simulink model "CryoDetXray"  (R2016b)
settings: Solver=ode45  StartTime=0.0  StopTime=10e-5  MaxStep=Tclk/4  RelTol=1e-3
values from neighbouring files (symbols this model uses):
  Fclk = Fadc    (= 307200000)    [setupCryoFPGAxray.m]
  Tclk = 1/Fclk    (= 3.25520833333e-09)    [setupCryoFPGAxray.m]
undefined symbols (not defined in the file or in its folder): AXI4, Lite, lpf, Naxi, xlipgetpartsetting
libraries: xbsIndex_r4 x1091, CryoDetLib x68, simulink x4, hdlsllib x1
(part 4 of 8)

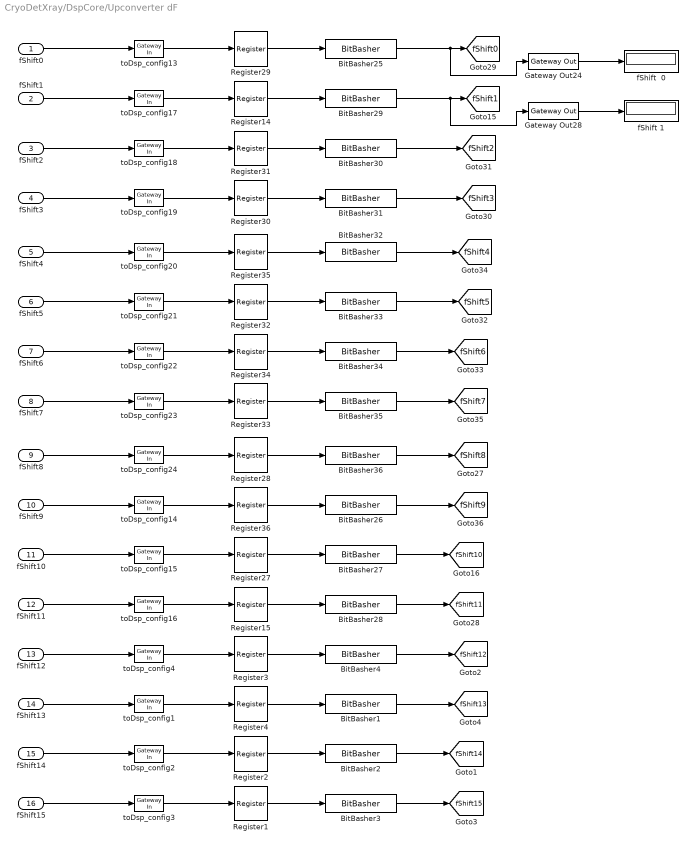
== system CryoDetXray/DspCore/Upconverter dF ==
  fShift0 : Inport
  fShift1 : Inport  Port=2
  fShift2 : Inport  Port=3
  fShift3 : Inport  Port=4
  fShift4 : Inport  Port=5
  fShift5 : Inport  Port=6
  fShift6 : Inport  Port=7
  fShift7 : Inport  Port=8
  fShift8 : Inport  Port=9
  fShift9 : Inport  Port=10
  fShift10 : Inport  Port=11
  fShift11 : Inport  Port=12
  fShift12 : Inport  Port=13
  fShift13 : Inport  Port=14
  fShift14 : Inport  Port=15
  fShift15 : Inport  Port=16
  BitBasher{1..4,25..36} (16 alike) : xbsIndex_r4/BitBasher  bitexpr=a={b[15:0]}  display_expr=on  sr_1=a  arith_type1=Unsigned  bin_pt1=16  sr_2=2  arith_type2=Unsigned  bin_pt2=0  sr_3=3  arith_type3=Unsigned  bin_pt3=0  sr_4=4  arith_type4=Unsigned  bin_pt4=0  dbl_ovrd=off  block_type=bitbasher
  Gateway Out24 : xbsIndex_r4/Gateway Out  inherit_from_input=on  hdl_port=off  rows=1  columns=1  UseAsDAC=off  DACChannel='1'  interface=None  automatic_assignment=on  address_offset=hex2dec('00')  intf_name=''  intf_description=''  timing_constraint=None  locs_specified=off  LOCs={}  io_standard={}  block_type=gatewayout
  Gateway Out28 : xbsIndex_r4/Gateway Out  inherit_from_input=on  hdl_port=off  rows=1  columns=1  UseAsDAC=off  DACChannel='1'  interface=None  automatic_assignment=on  address_offset=hex2dec('00')  intf_name=''  intf_description=''  timing_constraint=None  locs_specified=off  LOCs={}  io_standard={}  block_type=gatewayout
  Register{1..4,14..15,27..36} (16 alike) : xbsIndex_r4/Register  init=0  rst=off  en=off  dbl_ovrd=off  block_type=register
  fShift  0 : Display
  fShift 1 : Display
  toDsp_config1 : xbsIndex_r4/Gateway In  gui_display_data_type=Fixed-point  arith_type=Unsigned  n_bits=32  bin_pt=0  preci_type=Single  exp_width=8  frac_width=24  rows=1  columns=1  quantization=Truncate  overflow=Wrap  period=Tclk*Naxi  UseAsADC=off  ADCChannel='1'  interface=AXI4-Lite  automatic_assignment=off  address_offset=hex2dec('8B4')  intf_name=''  intf_description=''  default_value=0  timing_constraint=None  locs_specified=off  LOCs={}  io_standard={}  inherit_from_input=off  hdl_port=on  dbl_ovrd=off  block_type=gatewayin
  toDsp_config13 : xbsIndex_r4/Gateway In  gui_display_data_type=Fixed-point  arith_type=Unsigned  n_bits=32  bin_pt=0  preci_type=Single  exp_width=8  frac_width=24  rows=1  columns=1  quantization=Truncate  overflow=Wrap  period=Tclk*Naxi  UseAsADC=off  ADCChannel='1'  interface=AXI4-Lite  automatic_assignment=off  address_offset=hex2dec('880')  intf_name=''  intf_description=''  default_value=0  timing_constraint=None  locs_specified=off  LOCs={}  io_standard={}  inherit_from_input=off  hdl_port=on  dbl_ovrd=off  block_type=gatewayin
  toDsp_config14 : xbsIndex_r4/Gateway In  gui_display_data_type=Fixed-point  arith_type=Unsigned  n_bits=32  bin_pt=0  preci_type=Single  exp_width=8  frac_width=24  rows=1  columns=1  quantization=Truncate  overflow=Wrap  period=Tclk*Naxi  UseAsADC=off  ADCChannel='1'  interface=AXI4-Lite  automatic_assignment=off  address_offset=hex2dec('8A4')  intf_name=''  intf_description=''  default_value=0  timing_constraint=None  locs_specified=off  LOCs={}  io_standard={}  inherit_from_input=off  hdl_port=on  dbl_ovrd=off  block_type=gatewayin
  toDsp_config15 : xbsIndex_r4/Gateway In  gui_display_data_type=Fixed-point  arith_type=Unsigned  n_bits=32  bin_pt=0  preci_type=Single  exp_width=8  frac_width=24  rows=1  columns=1  quantization=Truncate  overflow=Wrap  period=Tclk*Naxi  UseAsADC=off  ADCChannel='1'  interface=AXI4-Lite  automatic_assignment=off  address_offset=hex2dec('8A8')  intf_name=''  intf_description=''  default_value=0  timing_constraint=None  locs_specified=off  LOCs={}  io_standard={}  inherit_from_input=off  hdl_port=on  dbl_ovrd=off  block_type=gatewayin
  toDsp_config16 : xbsIndex_r4/Gateway In  gui_display_data_type=Fixed-point  arith_type=Unsigned  n_bits=32  bin_pt=0  preci_type=Single  exp_width=8  frac_width=24  rows=1  columns=1  quantization=Truncate  overflow=Wrap  period=Tclk*Naxi  UseAsADC=off  ADCChannel='1'  interface=AXI4-Lite  automatic_assignment=off  address_offset=hex2dec('8AC')  intf_name=''  intf_description=''  default_value=0  timing_constraint=None  locs_specified=off  LOCs={}  io_standard={}  inherit_from_input=off  hdl_port=on  dbl_ovrd=off  block_type=gatewayin
  toDsp_config17 : xbsIndex_r4/Gateway In  gui_display_data_type=Fixed-point  arith_type=Unsigned  n_bits=32  bin_pt=0  preci_type=Single  exp_width=8  frac_width=24  rows=1  columns=1  quantization=Truncate  overflow=Wrap  period=Tclk*Naxi  UseAsADC=off  ADCChannel='1'  interface=AXI4-Lite  automatic_assignment=off  address_offset=hex2dec('884')  intf_name=''  intf_description=''  default_value=0  timing_constraint=None  locs_specified=off  LOCs={}  io_standard={}  inherit_from_input=off  hdl_port=on  dbl_ovrd=off  block_type=gatewayin
  toDsp_config18 : xbsIndex_r4/Gateway In  gui_display_data_type=Fixed-point  arith_type=Unsigned  n_bits=32  bin_pt=0  preci_type=Single  exp_width=8  frac_width=24  rows=1  columns=1  quantization=Truncate  overflow=Wrap  period=Tclk*Naxi  UseAsADC=off  ADCChannel='1'  interface=AXI4-Lite  automatic_assignment=off  address_offset=hex2dec('888')  intf_name=''  intf_description=''  default_value=0  timing_constraint=None  locs_specified=off  LOCs={}  io_standard={}  inherit_from_input=off  hdl_port=on  dbl_ovrd=off  block_type=gatewayin
  toDsp_config19 : xbsIndex_r4/Gateway In  gui_display_data_type=Fixed-point  arith_type=Unsigned  n_bits=32  bin_pt=0  preci_type=Single  exp_width=8  frac_width=24  rows=1  columns=1  quantization=Truncate  overflow=Wrap  period=Tclk*Naxi  UseAsADC=off  ADCChannel='1'  interface=AXI4-Lite  automatic_assignment=off  address_offset=hex2dec('88c')  intf_name=''  intf_description=''  default_value=0  timing_constraint=None  locs_specified=off  LOCs={}  io_standard={}  inherit_from_input=off  hdl_port=on  dbl_ovrd=off  block_type=gatewayin
  toDsp_config2 : xbsIndex_r4/Gateway In  gui_display_data_type=Fixed-point  arith_type=Unsigned  n_bits=32  bin_pt=0  preci_type=Single  exp_width=8  frac_width=24  rows=1  columns=1  quantization=Truncate  overflow=Wrap  period=Tclk*Naxi  UseAsADC=off  ADCChannel='1'  interface=AXI4-Lite  automatic_assignment=off  address_offset=hex2dec('8B8')  intf_name=''  intf_description=''  default_value=0  timing_constraint=None  locs_specified=off  LOCs={}  io_standard={}  inherit_from_input=off  hdl_port=on  dbl_ovrd=off  block_type=gatewayin
  toDsp_config20 : xbsIndex_r4/Gateway In  gui_display_data_type=Fixed-point  arith_type=Unsigned  n_bits=32  bin_pt=0  preci_type=Single  exp_width=8  frac_width=24  rows=1  columns=1  quantization=Truncate  overflow=Wrap  period=Tclk*Naxi  UseAsADC=off  ADCChannel='1'  interface=AXI4-Lite  automatic_assignment=off  address_offset=hex2dec('890')  intf_name=''  intf_description=''  default_value=0  timing_constraint=None  locs_specified=off  LOCs={}  io_standard={}  inherit_from_input=off  hdl_port=on  dbl_ovrd=off  block_type=gatewayin
  toDsp_config21 : xbsIndex_r4/Gateway In  gui_display_data_type=Fixed-point  arith_type=Unsigned  n_bits=32  bin_pt=0  preci_type=Single  exp_width=8  frac_width=24  rows=1  columns=1  quantization=Truncate  overflow=Wrap  period=Tclk*Naxi  UseAsADC=off  ADCChannel='1'  interface=AXI4-Lite  automatic_assignment=off  address_offset=hex2dec('894')  intf_name=''  intf_description=''  default_value=0  timing_constraint=None  locs_specified=off  LOCs={}  io_standard={}  inherit_from_input=off  hdl_port=on  dbl_ovrd=off  block_type=gatewayin
  toDsp_config22 : xbsIndex_r4/Gateway In  gui_display_data_type=Fixed-point  arith_type=Unsigned  n_bits=32  bin_pt=0  preci_type=Single  exp_width=8  frac_width=24  rows=1  columns=1  quantization=Truncate  overflow=Wrap  period=Tclk*Naxi  UseAsADC=off  ADCChannel='1'  interface=AXI4-Lite  automatic_assignment=off  address_offset=hex2dec('898')  intf_name=''  intf_description=''  default_value=0  timing_constraint=None  locs_specified=off  LOCs={}  io_standard={}  inherit_from_input=off  hdl_port=on  dbl_ovrd=off  block_type=gatewayin
  toDsp_config23 : xbsIndex_r4/Gateway In  gui_display_data_type=Fixed-point  arith_type=Unsigned  n_bits=32  bin_pt=0  preci_type=Single  exp_width=8  frac_width=24  rows=1  columns=1  quantization=Truncate  overflow=Wrap  period=Tclk*Naxi  UseAsADC=off  ADCChannel='1'  interface=AXI4-Lite  automatic_assignment=off  address_offset=hex2dec('89c')  intf_name=''  intf_description=''  default_value=0  timing_constraint=None  locs_specified=off  LOCs={}  io_standard={}  inherit_from_input=off  hdl_port=on  dbl_ovrd=off  block_type=gatewayin
  toDsp_config24 : xbsIndex_r4/Gateway In  gui_display_data_type=Fixed-point  arith_type=Unsigned  n_bits=32  bin_pt=0  preci_type=Single  exp_width=8  frac_width=24  rows=1  columns=1  quantization=Truncate  overflow=Wrap  period=Tclk*Naxi  UseAsADC=off  ADCChannel='1'  interface=AXI4-Lite  automatic_assignment=off  address_offset=hex2dec('8A0')  intf_name=''  intf_description=''  default_value=0  timing_constraint=None  locs_specified=off  LOCs={}  io_standard={}  inherit_from_input=off  hdl_port=on  dbl_ovrd=off  block_type=gatewayin
  toDsp_config3 : xbsIndex_r4/Gateway In  gui_display_data_type=Fixed-point  arith_type=Unsigned  n_bits=32  bin_pt=0  preci_type=Single  exp_width=8  frac_width=24  rows=1  columns=1  quantization=Truncate  overflow=Wrap  period=Tclk*Naxi  UseAsADC=off  ADCChannel='1'  interface=AXI4-Lite  automatic_assignment=off  address_offset=hex2dec('8BC')  intf_name=''  intf_description=''  default_value=0  timing_constraint=None  locs_specified=off  LOCs={}  io_standard={}  inherit_from_input=off  hdl_port=on  dbl_ovrd=off  block_type=gatewayin
  toDsp_config4 : xbsIndex_r4/Gateway In  gui_display_data_type=Fixed-point  arith_type=Unsigned  n_bits=32  bin_pt=0  preci_type=Single  exp_width=8  frac_width=24  rows=1  columns=1  quantization=Truncate  overflow=Wrap  period=Tclk*Naxi  UseAsADC=off  ADCChannel='1'  interface=AXI4-Lite  automatic_assignment=off  address_offset=hex2dec('8B0')  intf_name=''  intf_description=''  default_value=0  timing_constraint=None  locs_specified=off  LOCs={}  io_standard={}  inherit_from_input=off  hdl_port=on  dbl_ovrd=off  block_type=gatewayin
  tag scope: fShift0=global, fShift10=global, fShift11=global, fShift12=global, fShift13=global, fShift14=global, fShift15=global, fShift1=global, fShift2=global, fShift3=global, fShift4=global, fShift5=global, fShift6=global, fShift7=global, fShift8=global, fShift9=global
  wires:
  toDsp_config13/1 -> Register29/1
  fShift10/1 -> toDsp_config15/1
  toDsp_config15/1 -> Register27/1
  Register32/1 -> BitBasher33/1
  BitBasher28/1 -> [fShift11]
  Register15/1 -> BitBasher28/1
  toDsp_config21/1 -> Register32/1
  BitBasher32/1 -> [fShift4]
  Register27/1 -> BitBasher27/1
  BitBasher27/1 -> [fShift10]
  fShift0/1 -> toDsp_config13/1
  fShift7/1 -> toDsp_config23/1
  toDsp_config23/1 -> Register33/1
  Gateway Out24/1 -> fShift  0/1
  Register30/1 -> BitBasher31/1
  BitBasher30/1 -> [fShift2]
  BitBasher31/1 -> [fShift3]
  Register33/1 -> BitBasher35/1
  Register36/1 -> BitBasher26/1
  fShift2/1 -> toDsp_config18/1
  toDsp_config18/1 -> Register31/1
  BitBasher29/1 -> Gateway Out28/1, [fShift1]
  BitBasher34/1 -> [fShift6]
  toDsp_config17/1 -> Register14/1
  fShift1/1 -> toDsp_config17/1
  Register28/1 -> BitBasher36/1
  BitBasher33/1 -> [fShift5]
  BitBasher35/1 -> [fShift7]
  BitBasher25/1 -> Gateway Out24/1, [fShift0]
  fShift5/1 -> toDsp_config21/1
  BitBasher36/1 -> [fShift8]
  Register34/1 -> BitBasher34/1
  BitBasher26/1 -> [fShift9]
  fShift8/1 -> toDsp_config24/1
  toDsp_config24/1 -> Register28/1
  fShift6/1 -> toDsp_config22/1
  toDsp_config22/1 -> Register34/1
  fShift11/1 -> toDsp_config16/1
  toDsp_config16/1 -> Register15/1
  fShift9/1 -> toDsp_config14/1
  toDsp_config14/1 -> Register36/1
  Register29/1 -> BitBasher25/1
  Register35/1 -> BitBasher32/1
  toDsp_config20/1 -> Register35/1
  fShift4/1 -> toDsp_config20/1
  Register14/1 -> BitBasher29/1
  Gateway Out28/1 -> fShift 1/1
  Register31/1 -> BitBasher30/1
  fShift3/1 -> toDsp_config19/1
  toDsp_config19/1 -> Register30/1
  fShift14/1 -> toDsp_config2/1
  toDsp_config2/1 -> Register2/1
  BitBasher3/1 -> [fShift15]
  Register1/1 -> BitBasher3/1
  Register2/1 -> BitBasher2/1
  BitBasher2/1 -> [fShift14]
  Register4/1 -> BitBasher1/1
  Register3/1 -> BitBasher4/1
  BitBasher4/1 -> [fShift12]
  BitBasher1/1 -> [fShift13]
  fShift12/1 -> toDsp_config4/1
  toDsp_config4/1 -> Register3/1
  fShift15/1 -> toDsp_config3/1
  toDsp_config3/1 -> Register1/1
  fShift13/1 -> toDsp_config1/1
  toDsp_config1/1 -> Register4/1

== system CryoDetXray/DspCore/eta input ==
  note: Punt for now on ch 3-11
  Re eta 0 : Inport
  Im eta 0 : Inport  Port=2
  Re eta 1 : Inport  Port=3
  Im eta 1 : Inport  Port=4
  Re eta 2 : Inport  Port=5
  Im eta 2 : Inport  Port=6
  Constant : xbsIndex_r4/Constant  const=0  gui_display_data_type=Fixed-point  arith_type=Signed (2's comp)  n_bits=32  bin_pt=14  preci_type=Single  exp_width=8  frac_width=24  explicit_period=off  period=1  equ=P=C  opselect=C  inp2=PCIN>>17  opr=+  inp1=P  carry=CIN  dbl_ovrd=off  block_type=constant
  Gateway Out{36..41} (6 alike) : xbsIndex_r4/Gateway Out  inherit_from_input=on  hdl_port=off  rows=1  columns=1  UseAsDAC=off  DACChannel='1'  interface=None  automatic_assignment=on  address_offset=hex2dec('00')  intf_name=''  intf_description=''  timing_constraint=None  locs_specified=off  LOCs={}  io_standard={}  block_type=gatewayout
  Register{37..42} (6 alike) : xbsIndex_r4/Register  init=0  rst=off  en=off  dbl_ovrd=off  block_type=register
  im eta 0 : Display
  im eta 1 : Display
  im eta 2 : Display
  re eta 0 : Display
  re eta 1 : Display
  re eta 2 : Display
  toDsp_config25 : xbsIndex_r4/Gateway In  gui_display_data_type=Fixed-point  arith_type="Signed  (2's comp)"  n_bits=32  bin_pt=14  preci_type=Single  exp_width=8  frac_width=24  rows=1  columns=1  quantization=Truncate  overflow=Wrap  period=Tclk*Naxi  UseAsADC=off  ADCChannel='1'  interface=AXI4-Lite  automatic_assignment=off  address_offset=hex2dec('C00')  intf_name=''  intf_description=''  default_value=0  timing_constraint=None  locs_specified=off  LOCs={}  io_standard={}  inherit_from_input=off  hdl_port=on  dbl_ovrd=off  block_type=gatewayin
  toDsp_config26 : xbsIndex_r4/Gateway In  gui_display_data_type=Fixed-point  arith_type="Signed  (2's comp)"  n_bits=32  bin_pt=14  preci_type=Single  exp_width=8  frac_width=24  rows=1  columns=1  quantization=Truncate  overflow=Wrap  period=Tclk*Naxi  UseAsADC=off  ADCChannel='1'  interface=AXI4-Lite  automatic_assignment=off  address_offset=hex2dec('D00')  intf_name=''  intf_description=''  default_value=0  timing_constraint=None  locs_specified=off  LOCs={}  io_standard={}  inherit_from_input=off  hdl_port=on  dbl_ovrd=off  block_type=gatewayin
  toDsp_config27 : xbsIndex_r4/Gateway In  gui_display_data_type=Fixed-point  arith_type="Signed  (2's comp)"  n_bits=32  bin_pt=14  preci_type=Single  exp_width=8  frac_width=24  rows=1  columns=1  quantization=Truncate  overflow=Wrap  period=Tclk*Naxi  UseAsADC=off  ADCChannel='1'  interface=AXI4-Lite  automatic_assignment=off  address_offset=hex2dec('C04')  intf_name=''  intf_description=''  default_value=0  timing_constraint=None  locs_specified=off  LOCs={}  io_standard={}  inherit_from_input=off  hdl_port=on  dbl_ovrd=off  block_type=gatewayin
  toDsp_config28 : xbsIndex_r4/Gateway In  gui_display_data_type=Fixed-point  arith_type="Signed  (2's comp)"  n_bits=32  bin_pt=14  preci_type=Single  exp_width=8  frac_width=24  rows=1  columns=1  quantization=Truncate  overflow=Wrap  period=Tclk*Naxi  UseAsADC=off  ADCChannel='1'  interface=AXI4-Lite  automatic_assignment=off  address_offset=hex2dec('D04')  intf_name=''  intf_description=''  default_value=0  timing_constraint=None  locs_specified=off  LOCs={}  io_standard={}  inherit_from_input=off  hdl_port=on  dbl_ovrd=off  block_type=gatewayin
  toDsp_config29 : xbsIndex_r4/Gateway In  gui_display_data_type=Fixed-point  arith_type="Signed  (2's comp)"  n_bits=32  bin_pt=14  preci_type=Single  exp_width=8  frac_width=24  rows=1  columns=1  quantization=Truncate  overflow=Wrap  period=Tclk*Naxi  UseAsADC=off  ADCChannel='1'  interface=AXI4-Lite  automatic_assignment=off  address_offset=hex2dec('C08')  intf_name=''  intf_description=''  default_value=0  timing_constraint=None  locs_specified=off  LOCs={}  io_standard={}  inherit_from_input=off  hdl_port=on  dbl_ovrd=off  block_type=gatewayin
  toDsp_config30 : xbsIndex_r4/Gateway In  gui_display_data_type=Fixed-point  arith_type="Signed  (2's comp)"  n_bits=32  bin_pt=14  preci_type=Single  exp_width=8  frac_width=24  rows=1  columns=1  quantization=Truncate  overflow=Wrap  period=Tclk*Naxi  UseAsADC=off  ADCChannel='1'  interface=AXI4-Lite  automatic_assignment=off  address_offset=hex2dec('D08')  intf_name=''  intf_description=''  default_value=0  timing_constraint=None  locs_specified=off  LOCs={}  io_standard={}  inherit_from_input=off  hdl_port=on  dbl_ovrd=off  block_type=gatewayin
  tag scope: imEta0=global, imEta10=global, imEta11=global, imEta12=global, imEta13=global, imEta14=global, imEta15=global, imEta1=global, imEta2=global, imEta3=global, imEta4=global, imEta5=global, imEta6=global, imEta7=global, imEta8=global, imEta9=global, reEta0=global, reEta10=global, reEta11=global, reEta12=global, reEta13=global, reEta14=global, reEta15=global, reEta1=global, reEta2=global, reEta3=global, reEta4=global, reEta5=global, reEta6=global, reEta7=global, reEta8=global, reEta9=global
  wires:
  toDsp_config28/1 -> Register39/1
  Im eta 1/1 -> toDsp_config28/1
  Register40/1 -> Gateway Out38/1, [reEta1]
  Gateway Out39/1 -> im eta 1/1
  Re eta 2/1 -> toDsp_config29/1
  Gateway Out40/1 -> re eta 2/1
  Register41/1 -> Gateway Out41/1, [imEta2]
  toDsp_config30/1 -> Register41/1
  Im eta 2/1 -> toDsp_config30/1
  toDsp_config27/1 -> Register40/1
  Re eta 1/1 -> toDsp_config27/1
  Gateway Out38/1 -> re eta 1/1
  Register39/1 -> Gateway Out39/1, [imEta1]
  Register42/1 -> Gateway Out40/1, [reEta2]
  Gateway Out41/1 -> im eta 2/1
  toDsp_config29/1 -> Register42/1
  Constant/1 -> [reEta4], [reEta5], [reEta6], [reEta7], [reEta8], [reEta9], [imEta9], [imEta10], [imEta12], [imEta13], [imEta14], [imEta15], [imEta11], [imEta8], [imEta7], [imEta6], [imEta5], [imEta4], [imEta3], [reEta15], [reEta14], [reEta13], [reEta12], [reEta11], [reEta10], [reEta3]
  toDsp_config25/1 -> Register38/1
  Re eta 0/1 -> toDsp_config25/1
  Gateway Out36/1 -> re eta 0/1
  Register37/1 -> Gateway Out37/1, [imEta0]
  toDsp_config26/1 -> Register37/1
  Im eta 0/1 -> toDsp_config26/1
  Register38/1 -> Gateway Out36/1, [reEta0]
  Gateway Out37/1 -> im eta 0/1

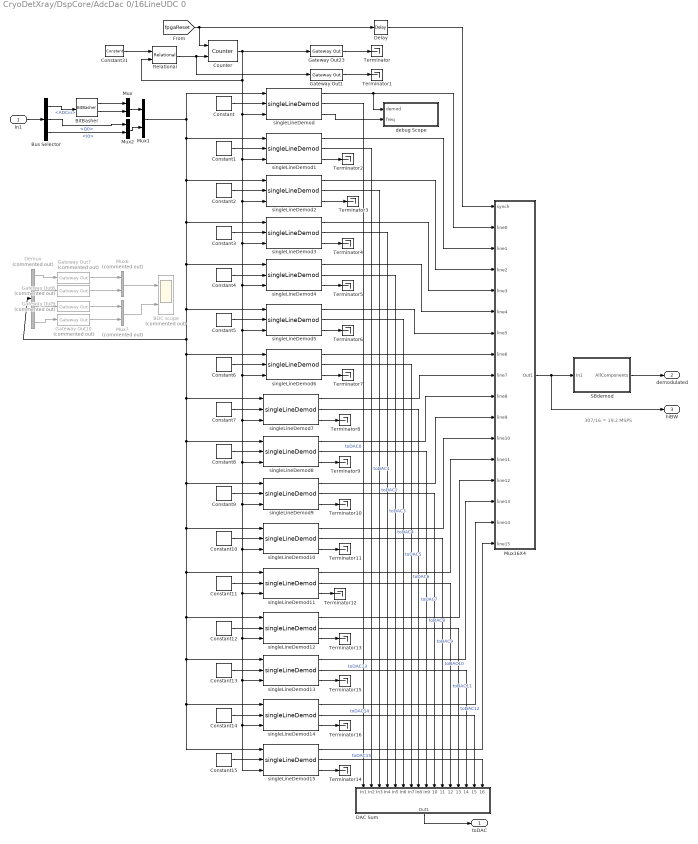
== system CryoDetXray/DspCore/AdcDac 0/16LineUDC 0 ==
  note: 307/16 = 19.2 MSPS
  In1 : Inport
  BDC scope : Scope  Commented=on  NumInputPorts=2
  BitBasher : xbsIndex_r4/BitBasher  bitexpr=|  display_expr=off  sr_1=Q  arith_type1="Signed  (2's comp)"  bin_pt1=15  sr_2=I  arith_type2="Signed  (2's comp)"  bin_pt2=15  sr_3=I  arith_type3=Unsigned  bin_pt3=0  sr_4=4  arith_type4=Unsigned  bin_pt4=0  dbl_ovrd=off  block_type=bitbasher
      | Q = {adc[15:0]}
      | I = {adc[31:16]}
  Bus Selector : BusSelector  OutputSignals=ADCin,refDel.Q0,refDel.I0
  Constant : xbsIndex_r4/Constant  const=0  gui_display_data_type=Fixed-point  arith_type=Unsigned  n_bits=4  bin_pt=0  preci_type=Single  exp_width=8  frac_width=24  explicit_period=off  period=1  equ=P=C  opselect=C  inp2=PCIN>>17  opr=+  inp1=P  carry=CIN  dbl_ovrd=off  block_type=constant
  Constant1 : xbsIndex_r4/Constant  const=1  gui_display_data_type=Fixed-point  arith_type=Unsigned  n_bits=4  bin_pt=0  preci_type=Single  exp_width=8  frac_width=24  explicit_period=off  period=1  equ=P=C  opselect=C  inp2=PCIN>>17  opr=+  inp1=P  carry=CIN  dbl_ovrd=off  block_type=constant
  Constant10 : xbsIndex_r4/Constant  const=10  gui_display_data_type=Fixed-point  arith_type=Unsigned  n_bits=4  bin_pt=0  preci_type=Single  exp_width=8  frac_width=24  explicit_period=off  period=1  equ=P=C  opselect=C  inp2=PCIN>>17  opr=+  inp1=P  carry=CIN  dbl_ovrd=off  block_type=constant
  Constant11 : xbsIndex_r4/Constant  const=11  gui_display_data_type=Fixed-point  arith_type=Unsigned  n_bits=4  bin_pt=0  preci_type=Single  exp_width=8  frac_width=24  explicit_period=off  period=1  equ=P=C  opselect=C  inp2=PCIN>>17  opr=+  inp1=P  carry=CIN  dbl_ovrd=off  block_type=constant
  Constant12 : xbsIndex_r4/Constant  const=12  gui_display_data_type=Fixed-point  arith_type=Unsigned  n_bits=4  bin_pt=0  preci_type=Single  exp_width=8  frac_width=24  explicit_period=off  period=1  equ=P=C  opselect=C  inp2=PCIN>>17  opr=+  inp1=P  carry=CIN  dbl_ovrd=off  block_type=constant
  Constant13 : xbsIndex_r4/Constant  const=13  gui_display_data_type=Fixed-point  arith_type=Unsigned  n_bits=4  bin_pt=0  preci_type=Single  exp_width=8  frac_width=24  explicit_period=off  period=1  equ=P=C  opselect=C  inp2=PCIN>>17  opr=+  inp1=P  carry=CIN  dbl_ovrd=off  block_type=constant
  Constant14 : xbsIndex_r4/Constant  const=14  gui_display_data_type=Fixed-point  arith_type=Unsigned  n_bits=4  bin_pt=0  preci_type=Single  exp_width=8  frac_width=24  explicit_period=off  period=1  equ=P=C  opselect=C  inp2=PCIN>>17  opr=+  inp1=P  carry=CIN  dbl_ovrd=off  block_type=constant
  Constant15 : xbsIndex_r4/Constant  const=15  gui_display_data_type=Fixed-point  arith_type=Unsigned  n_bits=4  bin_pt=0  preci_type=Single  exp_width=8  frac_width=24  explicit_period=off  period=1  equ=P=C  opselect=C  inp2=PCIN>>17  opr=+  inp1=P  carry=CIN  dbl_ovrd=off  block_type=constant
  Constant2 : xbsIndex_r4/Constant  const=2  gui_display_data_type=Fixed-point  arith_type=Unsigned  n_bits=4  bin_pt=0  preci_type=Single  exp_width=8  frac_width=24  explicit_period=off  period=1  equ=P=C  opselect=C  inp2=PCIN>>17  opr=+  inp1=P  carry=CIN  dbl_ovrd=off  block_type=constant
  Constant3 : xbsIndex_r4/Constant  const=3  gui_display_data_type=Fixed-point  arith_type=Unsigned  n_bits=4  bin_pt=0  preci_type=Single  exp_width=8  frac_width=24  explicit_period=off  period=1  equ=P=C  opselect=C  inp2=PCIN>>17  opr=+  inp1=P  carry=CIN  dbl_ovrd=off  block_type=constant
  Constant31 : xbsIndex_r4/Constant  const=31  gui_display_data_type=Fixed-point  arith_type=Unsigned  n_bits=5  bin_pt=0  preci_type=Single  exp_width=8  frac_width=24  explicit_period=off  period=1  equ=P=C  opselect=C  inp2=PCIN>>17  opr=+  inp1=P  carry=CIN  dbl_ovrd=off  block_type=constant
  Constant4 : xbsIndex_r4/Constant  const=4  gui_display_data_type=Fixed-point  arith_type=Unsigned  n_bits=4  bin_pt=0  preci_type=Single  exp_width=8  frac_width=24  explicit_period=off  period=1  equ=P=C  opselect=C  inp2=PCIN>>17  opr=+  inp1=P  carry=CIN  dbl_ovrd=off  block_type=constant
  Constant5 : xbsIndex_r4/Constant  const=5  gui_display_data_type=Fixed-point  arith_type=Unsigned  n_bits=4  bin_pt=0  preci_type=Single  exp_width=8  frac_width=24  explicit_period=off  period=1  equ=P=C  opselect=C  inp2=PCIN>>17  opr=+  inp1=P  carry=CIN  dbl_ovrd=off  block_type=constant
  Constant6 : xbsIndex_r4/Constant  const=6  gui_display_data_type=Fixed-point  arith_type=Unsigned  n_bits=4  bin_pt=0  preci_type=Single  exp_width=8  frac_width=24  explicit_period=off  period=1  equ=P=C  opselect=C  inp2=PCIN>>17  opr=+  inp1=P  carry=CIN  dbl_ovrd=off  block_type=constant
  Constant7 : xbsIndex_r4/Constant  const=7  gui_display_data_type=Fixed-point  arith_type=Unsigned  n_bits=4  bin_pt=0  preci_type=Single  exp_width=8  frac_width=24  explicit_period=off  period=1  equ=P=C  opselect=C  inp2=PCIN>>17  opr=+  inp1=P  carry=CIN  dbl_ovrd=off  block_type=constant
  Constant8 : xbsIndex_r4/Constant  const=8  gui_display_data_type=Fixed-point  arith_type=Unsigned  n_bits=4  bin_pt=0  preci_type=Single  exp_width=8  frac_width=24  explicit_period=off  period=1  equ=P=C  opselect=C  inp2=PCIN>>17  opr=+  inp1=P  carry=CIN  dbl_ovrd=off  block_type=constant
  Constant9 : xbsIndex_r4/Constant  const=9  gui_display_data_type=Fixed-point  arith_type=Unsigned  n_bits=4  bin_pt=0  preci_type=Single  exp_width=8  frac_width=24  explicit_period=off  period=1  equ=P=C  opselect=C  inp2=PCIN>>17  opr=+  inp1=P  carry=CIN  dbl_ovrd=off  block_type=constant
  Counter : xbsIndex_r4/Counter  cnt_type=Count Limited  cnt_to=31  operation=Up  start_count=0  cnt_by_val=1  arith_type=Unsigned  n_bits=5  bin_pt=0  load_pin=off  rst=on  en=on  explicit_period=off  period=Tclk  use_behavioral_HDL=off  implementation=Fabric  dbl_ovrd=off  block_type=counter
  DAC Sum : Subsystem
  Delay : xbsIndex_r4/Delay  rst=off  infoeditControl=Selection of Reset will increase slice count due to use of real FFs and instead of SRLs  en=off  latency=6  reg_retiming=off  dbl_ovrd=off  block_type=delay
  Demux : Demux  Commented=on
  Gateway Out1 : xbsIndex_r4/Gateway Out  inherit_from_input=off  hdl_port=off  rows=1  columns=1  UseAsDAC=off  DACChannel='1'  interface=None  automatic_assignment=on  address_offset=hex2dec('00')  intf_name=''  intf_description=''  timing_constraint=None  locs_specified=off  LOCs={}  io_standard={}  block_type=gatewayout
  Gateway Out{7..10} (4 alike) : xbsIndex_r4/Gateway Out  Commented=on  inherit_from_input=off  hdl_port=off  rows=1  columns=1  UseAsDAC=off  DACChannel='1'  interface=None  automatic_assignment=on  address_offset=hex2dec('00')  intf_name=''  intf_description=''  timing_constraint=None  locs_specified=off  LOCs={}  io_standard={}  block_type=gatewayout
  Gateway Out23 : xbsIndex_r4/Gateway Out  inherit_from_input=off  hdl_port=off  rows=1  columns=1  UseAsDAC=off  DACChannel='1'  interface=None  automatic_assignment=on  address_offset=hex2dec('00')  intf_name=''  intf_description=''  timing_constraint=None  locs_specified=off  LOCs={}  io_standard={}  block_type=gatewayout
  Mux : Mux  Inputs=2
  Mux1 : Mux  Inputs=2
  Mux16X4 : Subsystem
  Mux2 : Mux  Inputs=2
  Mux6 : Mux  Commented=on  Inputs=2
  Mux7 : Mux  Commented=on  Inputs=2
  Relational : xbsIndex_r4/Relational  mode=a!=b  op_type=Bool  en=off  latency=0  dbl_ovrd=off  block_type=relational
  SBdemod : Subsystem
  Terminator{,1..16} (17 alike) : Terminator
  debug Scope : Subsystem
  singleLineDemod{,1..15} (16 alike) : CryoDetLib/singleLineDemod
  toDAC : Outport
  demodulated : Outport  Port=2
  hiBW : Outport  Port=3
  wires:
  [fpgaReset] -> Counter/1, Delay/1
  singleLineDemod7/1 -> Mux16X4/9(line7)
  singleLineDemod6/1 -> Mux16X4/8(line6)
  singleLineDemod5/1 -> Mux16X4/7(line5)
  singleLineDemod4/1 -> Mux16X4/6(line4)
  singleLineDemod3/1 -> Mux16X4/5(line3)
  singleLineDemod2/1 -> Mux16X4/4(line2)
  Mux16X4/1(Out1) -> hiBW/1, SBdemod/1(In1)
  singleLineDemod1/1 -> Mux16X4/3(line1)
  singleLineDemod/1 -> debug Scope/1(demod), Mux16X4/2(line0)
  singleLineDemod8/1 -> Mux16X4/10(line8)
  singleLineDemod9/1 -> Mux16X4/11(line9)
  singleLineDemod10/1 -> Mux16X4/12(line10)
  singleLineDemod11/1 -> Mux16X4/13(line11)
  singleLineDemod11/2 -> DAC Sum/12(In12)  "toDAC11"
  singleLineDemod10/2 -> DAC Sum/11(In11)  "toDAC10"
  singleLineDemod9/2 -> DAC Sum/10(In10)  "toDAC9"
  singleLineDemod8/2 -> DAC Sum/9(In9)  "toDAC8"
  singleLineDemod7/2 -> DAC Sum/8(In8)  "toDAC7"
  singleLineDemod6/2 -> DAC Sum/7(In7)  "toDAC6"
  singleLineDemod5/2 -> DAC Sum/6(In6)  "toDAC5"
  singleLineDemod4/2 -> DAC Sum/5(In5)  "toDAC4"
  singleLineDemod3/2 -> DAC Sum/4(In4)  "toDAC3"
  singleLineDemod2/2 -> DAC Sum/3(In3)  "toDAC2"
  singleLineDemod1/2 -> DAC Sum/2(In2)  "toDAC1"
  singleLineDemod/2 -> DAC Sum/1(In1)  "toDAC0"
  SBdemod/1(AllComponents) -> demodulated/1
  Gateway Out10/1 -> Mux7/2
  Gateway Out9/1 -> Mux7/1
  Gateway Out8/1 -> Mux6/2
  Gateway Out7/1 -> Mux6/1
  Mux6/1 -> BDC scope/1
  Mux7/1 -> BDC scope/2
  Demux/1 -> Gateway Out7/1
  Demux/4 -> Gateway Out10/1
  Demux/3 -> Gateway Out9/1
  Demux/2 -> Gateway Out8/1
  Delay/1 -> Mux16X4/1(synch)
  Constant/1 -> singleLineDemod/2
  Constant1/1 -> singleLineDemod1/2
  Constant2/1 -> singleLineDemod2/2
  Constant3/1 -> singleLineDemod3/2
  Constant4/1 -> singleLineDemod4/2
  Constant5/1 -> singleLineDemod5/2
  Constant6/1 -> singleLineDemod6/2
  Constant7/1 -> singleLineDemod7/2
  Constant8/1 -> singleLineDemod8/2
  Constant9/1 -> singleLineDemod9/2
  Constant10/1 -> singleLineDemod10/2
  Constant11/1 -> singleLineDemod11/2
  Gateway Out23/1 -> Terminator/1
  Gateway Out1/1 -> Terminator1/1
  Relational/1 -> Gateway Out1/1, Counter/2
  Constant31/1 -> Relational/1
  Constant12/1 -> singleLineDemod12/2
  Constant13/1 -> singleLineDemod13/2
  Constant14/1 -> singleLineDemod14/2
  Constant15/1 -> singleLineDemod15/2
  Counter/1 -> Gateway Out23/1, Relational/2, singleLineDemod2/3, singleLineDemod3/3, singleLineDemod10/3, singleLineDemod11/3, singleLineDemod12/3, singleLineDemod15/3, singleLineDemod14/3, singleLineDemod13/3, singleLineDemod9/3, singleLineDemod8/3, singleLineDemod7/3, singleLineDemod6/3, singleLineDemod5/3, singleLineDemod4/3, singleLineDemod1/3, singleLineDemod/3
  singleLineDemod12/1 -> Mux16X4/14(line12)
  singleLineDemod12/2 -> DAC Sum/13(In13)  "toDAC12"
  singleLineDemod13/1 -> Mux16X4/15(line13)
  singleLineDemod13/2 -> DAC Sum/14(In14)  "toDAC13"
  singleLineDemod14/1 -> Mux16X4/16(line14)
  singleLineDemod14/2 -> DAC Sum/15(In15)  "toDAC14"
  singleLineDemod15/1 -> Mux16X4/17(line15)
  singleLineDemod15/2 -> DAC Sum/16(In16)  "toDAC15"
  BitBasher/1 -> Mux/1
  BitBasher/2 -> Mux/2
  Mux1/1 -> singleLineDemod/1, singleLineDemod1/1, singleLineDemod2/1, singleLineDemod3/1, singleLineDemod4/1, singleLineDemod5/1, singleLineDemod6/1, singleLineDemod7/1, singleLineDemod8/1, singleLineDemod9/1, singleLineDemod10/1, singleLineDemod11/1, singleLineDemod12/1, singleLineDemod13/1, singleLineDemod14/1, singleLineDemod15/1, Demux/1
  In1/1 -> Bus Selector/1
  Bus Selector/1 -> BitBasher/1  "<ADCin>"
  Mux/1 -> Mux1/1
  DAC Sum/1(Out1) -> toDAC/1
  Mux2/1 -> Mux1/2
  Bus Selector/2 -> Mux2/1  "<Q0>"
  Bus Selector/3 -> Mux2/2  "<I0>"
  singleLineDemod/3 -> debug Scope/2(freq)
  singleLineDemod1/3 -> Terminator2/1
  singleLineDemod2/3 -> Terminator3/1
  singleLineDemod3/3 -> Terminator4/1
  singleLineDemod4/3 -> Terminator5/1
  singleLineDemod5/3 -> Terminator6/1
  singleLineDemod6/3 -> Terminator7/1
  singleLineDemod7/3 -> Terminator8/1
  singleLineDemod8/3 -> Terminator9/1
  singleLineDemod9/3 -> Terminator10/1
  singleLineDemod10/3 -> Terminator11/1
  singleLineDemod11/3 -> Terminator12/1
  singleLineDemod12/3 -> Terminator13/1
  singleLineDemod15/3 -> Terminator14/1
  singleLineDemod13/3 -> Terminator15/1
  singleLineDemod14/3 -> Terminator16/1

== system CryoDetXray/DspCore/AdcDac 0/16LineUDC 1 ==
  note: Null for now, eventually copy twelveLineUDC 0
      | when we need more than 16 lines per ADC channel
  In1 : Inport
  Out1 : Outport
  wires:
  In1/1 -> Out1/1

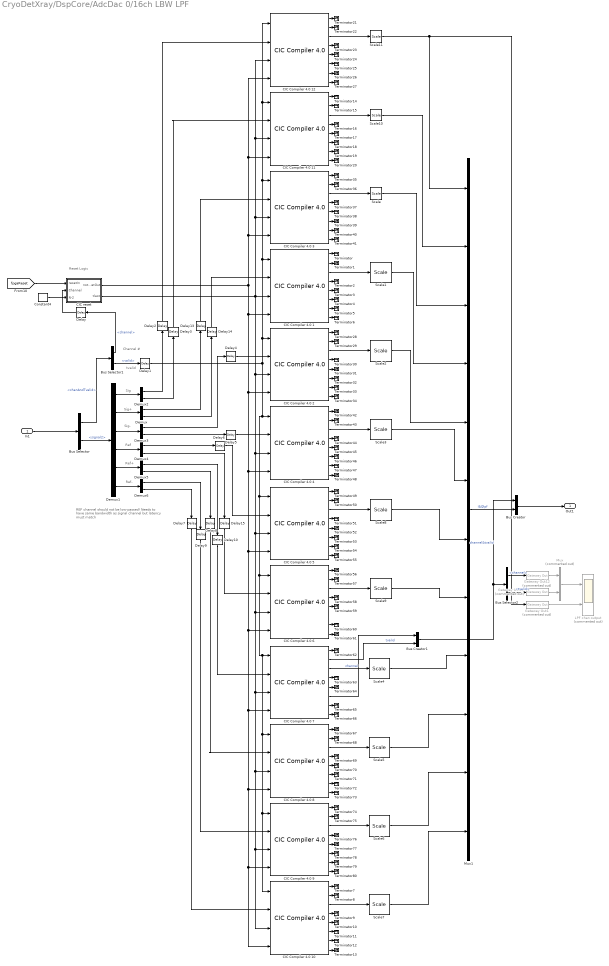
== system CryoDetXray/DspCore/AdcDac 0/16ch LBW LPF ==
  note: Reset Logic
  note: REF channel should not be low-passed!
      | Needs to have same bandwidth as signal channel
      | but latency must match
  note: tvalid
  note: Channel #
  note: Sig+
  note: Sig-
  note: Ref+
  note: Ref
  note: Sig
  note: Ref-
  In1 : Inport
  Bus Creator : BusCreator  Inputs=2
  Bus Creator1 : BusCreator  Inputs=2
  Bus Selector : BusSelector  OutputSignals=chanAndTvalid,signal2
  Bus Selector1 : BusSelector  OutputSignals=channel,valid
  Bus Selector2 : BusSelector  OutputSignals=channel,tvalid
  CIC Compiler 4.0 {1..12} (12 alike) : xbsIndex_r4/CIC Compiler 4.0   filter_type=Decimation  number_of_stages=3  differential_delay=1  number_of_channels=16  sample_rate_changes=Fixed  fixed_or_initial_rate=8  minimum_rate=8  maximum_rate=8  ratespecification=Sample_Period  sampleperiod=1  hardwareoversamplingrate=1  quantization=Truncation  output_data_width=24  use_xtreme_dsp_slice=off  use_streaming_interface=off  has_aclken=off  has_aresetn=on  has_dout_tready=off  trim_axipin_name=on  gui_behaviour=Sysgen_GUI  input_data_width=18  ip_name=CIC Compiler  ip_version=4.0  dsptool_ready=true  wrapper_available=true  port_translation_map={ 'aclken' => 'en', 'aresetn' => 'rst' }  ipcore_xco_need_fpga_part=true  ipcore_verbose=false  block_type=cic_compiler_v4_0
  CIC reset : Subsystem
  Constant4 : xbsIndex_r4/Constant  const=14  gui_display_data_type=Fixed-point  arith_type=Unsigned  n_bits=4  bin_pt=0  preci_type=Single  exp_width=8  frac_width=24  explicit_period=off  period=1  equ=P=C  opselect=C  inp2=PCIN>>17  opr=+  inp1=P  carry=CIN  dbl_ovrd=off  block_type=constant
  Delay{,1..10,13..15} (14 alike) : xbsIndex_r4/Delay  rst=off  infoeditControl=Selection of Reset will increase slice count due to use of real FFs and instead of SRLs  en=off  latency=1  reg_retiming=on  dbl_ovrd=off  block_type=delay
  Demux{,2..6} (6 alike) : Demux  Outputs=2
  Demux1 : Demux  Outputs=6
  Gateway Out1 : xbsIndex_r4/Gateway Out  Commented=on  inherit_from_input=off  hdl_port=off  rows=1  columns=1  UseAsDAC=off  DACChannel='1'  interface=None  automatic_assignment=on  address_offset=hex2dec('00')  intf_name=''  intf_description=''  timing_constraint=None  locs_specified=off  LOCs={}  io_standard={}  block_type=gatewayout
  Gateway Out12 : xbsIndex_r4/Gateway Out  Commented=on  inherit_from_input=off  hdl_port=off  rows=1  columns=1  UseAsDAC=off  DACChannel='1'  interface=None  automatic_assignment=on  address_offset=hex2dec('00')  intf_name=''  intf_description=''  timing_constraint=None  locs_specified=off  LOCs={}  io_standard={}  block_type=gatewayout
  Gateway Out13 : xbsIndex_r4/Gateway Out  Commented=on  inherit_from_input=off  hdl_port=off  rows=1  columns=1  UseAsDAC=off  DACChannel='1'  interface=None  automatic_assignment=on  address_offset=hex2dec('00')  intf_name=''  intf_description=''  timing_constraint=None  locs_specified=off  LOCs={}  io_standard={}  block_type=gatewayout
  LPF chan output : Scope  Commented=on  NumInputPorts=2
  Mux : Mux  Commented=on  Inputs=2
  Mux1 : Mux  Inputs=12
  Scale{,1..11} (12 alike) : xbsIndex_r4/Scale  scale_factor=-9  dbl_ovrd=off  block_type=scale
  Terminator{,1..80} (81 alike) : Terminator
  Out1 : Outport
  wires:
  Demux1/1 -> Demux2/1
  Demux1/2 -> Demux/1
  Demux1/3 -> Demux3/1
  Demux1/5 -> Demux5/1
  Demux1/6 -> Demux6/1
  Bus Selector/2 -> Demux1/1  "<signal2>"
  In1/1 -> Bus Selector/1
  Demux1/4 -> Demux4/1
  Demux/1 -> Delay13/1
  Demux/2 -> Delay14/1
  Demux3/1 -> Delay4/1
  Demux3/2 -> Delay5/1
  Demux5/1 -> Delay10/1
  Demux5/2 -> Delay8/1
  Demux6/1 -> Delay9/1
  Demux6/2 -> Delay7/1
  Bus Selector1/2 -> Delay1/1  "<valid>"
  Bus Selector1/1 -> Delay/1  "<channel>"
  Bus Selector/1 -> Bus Selector1/1  "<chanAndTvalid>"
  CIC Compiler 4.0 3/3 -> Scale/1
  CIC Compiler 4.0 1/3 -> Scale1/1
  CIC Compiler 4.0 2/3 -> Scale2/1
  CIC Compiler 4.0 4/3 -> Scale3/1
  Demux4/1 -> Delay6/1
  Demux4/2 -> Delay15/1
  CIC Compiler 4.0 7/3 -> Scale4/1
  CIC Compiler 4.0 8/3 -> Scale5/1
  CIC Compiler 4.0 9/3 -> Scale6/1
  CIC Compiler 4.0 10/3 -> Scale7/1
  Mux1/1 -> Bus Creator/2  "I&Qlpf"
  Bus Creator/1 -> Out1/1
  Bus Creator1/1 -> Bus Creator/1, Bus Selector2/1  "channel&tvalid"
  CIC Compiler 4.0 7/2 -> Bus Creator1/2  "tvalid"
  CIC Compiler 4.0 7/6 -> Bus Creator1/1  "channel"
  CIC reset/1(notResetOut) -> CIC Compiler 4.0 11/4, CIC Compiler 4.0 12/4, CIC Compiler 4.0 3/4, CIC Compiler 4.0 1/4, CIC Compiler 4.0 2/4, CIC Compiler 4.0 4/4, CIC Compiler 4.0 5/4, CIC Compiler 4.0 6/4, CIC Compiler 4.0 7/4, CIC Compiler 4.0 8/4, CIC Compiler 4.0 9/4, CIC Compiler 4.0 10/4
  Constant4/1 -> CIC reset/3(N-2)
  [fpgaReset] -> CIC reset/1(resetIn)
  CIC reset/2(tlast) -> CIC Compiler 4.0 11/3, CIC Compiler 4.0 12/3, CIC Compiler 4.0 3/3, CIC Compiler 4.0 2/3, CIC Compiler 4.0 5/3, CIC Compiler 4.0 6/3, CIC Compiler 4.0 8/3, CIC Compiler 4.0 9/3, CIC Compiler 4.0 10/3, CIC Compiler 4.0 7/3, CIC Compiler 4.0 4/3, CIC Compiler 4.0 1/3
  Bus Selector2/2 -> Gateway Out13/1  "<tvalid>"
  Bus Selector2/1 -> Gateway Out12/1  "<channel>"
  Gateway Out12/1 -> Mux/1
  Gateway Out13/1 -> Mux/2
  Mux/1 -> LPF chan output/1
  CIC Compiler 4.0 5/3 -> Scale8/1
  CIC Compiler 4.0 6/3 -> Scale9/1
  Demux2/2 -> Delay3/1
  Demux2/1 -> Delay2/1
  Scale7/1 -> Mux1/12
  Scale6/1 -> Mux1/11
  Scale5/1 -> Mux1/10
  Scale4/1 -> Mux1/9
  Scale9/1 -> Mux1/8
  Scale8/1 -> Mux1/7
  Scale3/1 -> Mux1/6
  Scale2/1 -> Mux1/5
  Scale1/1 -> Mux1/4
  Scale/1 -> Mux1/3
  CIC Compiler 4.0 11/3 -> Scale10/1
  CIC Compiler 4.0 12/3 -> Scale11/1
  Scale11/1 -> Gateway Out1/1, Mux1/1
  Scale10/1 -> Mux1/2
  CIC Compiler 4.0 1/1 -> Terminator/1
  CIC Compiler 4.0 1/2 -> Terminator1/1
  CIC Compiler 4.0 1/4 -> Terminator2/1
  CIC Compiler 4.0 1/5 -> Terminator3/1
  CIC Compiler 4.0 1/6 -> Terminator4/1
  CIC Compiler 4.0 1/7 -> Terminator5/1
  CIC Compiler 4.0 1/8 -> Terminator6/1
  CIC Compiler 4.0 10/1 -> Terminator7/1
  CIC Compiler 4.0 10/2 -> Terminator8/1
  CIC Compiler 4.0 10/4 -> Terminator9/1
  CIC Compiler 4.0 10/5 -> Terminator10/1
  CIC Compiler 4.0 10/6 -> Terminator11/1
  CIC Compiler 4.0 10/7 -> Terminator12/1
  CIC Compiler 4.0 10/8 -> Terminator13/1
  CIC Compiler 4.0 11/1 -> Terminator14/1
  CIC Compiler 4.0 11/2 -> Terminator15/1
  CIC Compiler 4.0 11/4 -> Terminator16/1
  CIC Compiler 4.0 11/5 -> Terminator17/1
  CIC Compiler 4.0 11/6 -> Terminator18/1
  CIC Compiler 4.0 11/7 -> Terminator19/1
  CIC Compiler 4.0 11/8 -> Terminator20/1
  CIC Compiler 4.0 12/1 -> Terminator21/1
  CIC Compiler 4.0 12/2 -> Terminator22/1
  CIC Compiler 4.0 12/4 -> Terminator23/1
  CIC Compiler 4.0 12/5 -> Terminator24/1
  CIC Compiler 4.0 12/6 -> Terminator25/1
  CIC Compiler 4.0 12/7 -> Terminator26/1
  CIC Compiler 4.0 12/8 -> Terminator27/1
  CIC Compiler 4.0 2/1 -> Terminator28/1
  CIC Compiler 4.0 2/2 -> Terminator29/1
  CIC Compiler 4.0 2/4 -> Terminator30/1
  CIC Compiler 4.0 2/5 -> Terminator31/1
  CIC Compiler 4.0 2/6 -> Terminator32/1
  CIC Compiler 4.0 2/7 -> Terminator33/1
  CIC Compiler 4.0 2/8 -> Terminator34/1
  CIC Compiler 4.0 3/1 -> Terminator35/1
  CIC Compiler 4.0 3/2 -> Terminator36/1
  CIC Compiler 4.0 3/4 -> Terminator37/1
  CIC Compiler 4.0 3/5 -> Terminator38/1
  CIC Compiler 4.0 3/6 -> Terminator39/1
  CIC Compiler 4.0 3/7 -> Terminator40/1
  CIC Compiler 4.0 3/8 -> Terminator41/1
  CIC Compiler 4.0 4/1 -> Terminator42/1
  CIC Compiler 4.0 4/2 -> Terminator43/1
  CIC Compiler 4.0 4/4 -> Terminator44/1
  CIC Compiler 4.0 4/5 -> Terminator45/1
  CIC Compiler 4.0 4/6 -> Terminator46/1
  CIC Compiler 4.0 4/7 -> Terminator47/1
  CIC Compiler 4.0 4/8 -> Terminator48/1
  CIC Compiler 4.0 5/1 -> Terminator49/1
  CIC Compiler 4.0 5/2 -> Terminator50/1
  CIC Compiler 4.0 5/4 -> Terminator51/1
  CIC Compiler 4.0 5/5 -> Terminator52/1
  CIC Compiler 4.0 5/6 -> Terminator53/1
  CIC Compiler 4.0 5/7 -> Terminator54/1
  CIC Compiler 4.0 5/8 -> Terminator55/1
  CIC Compiler 4.0 6/1 -> Terminator56/1
  CIC Compiler 4.0 6/2 -> Terminator57/1
  CIC Compiler 4.0 6/4 -> Terminator58/1
  CIC Compiler 4.0 6/5 -> Terminator59/1
  CIC Compiler 4.0 6/7 -> Terminator60/1
  CIC Compiler 4.0 6/8 -> Terminator61/1
  CIC Compiler 4.0 7/1 -> Terminator62/1
  CIC Compiler 4.0 7/4 -> Terminator63/1
  CIC Compiler 4.0 7/5 -> Terminator64/1
  CIC Compiler 4.0 7/7 -> Terminator65/1
  CIC Compiler 4.0 7/8 -> Terminator66/1
  CIC Compiler 4.0 8/1 -> Terminator67/1
  CIC Compiler 4.0 8/2 -> Terminator68/1
  CIC Compiler 4.0 8/4 -> Terminator69/1
  CIC Compiler 4.0 8/5 -> Terminator70/1
  CIC Compiler 4.0 8/6 -> Terminator71/1
  CIC Compiler 4.0 8/7 -> Terminator72/1
  CIC Compiler 4.0 8/8 -> Terminator73/1
  CIC Compiler 4.0 9/1 -> Terminator74/1
  CIC Compiler 4.0 9/2 -> Terminator75/1
  CIC Compiler 4.0 9/4 -> Terminator76/1
  CIC Compiler 4.0 9/5 -> Terminator77/1
  CIC Compiler 4.0 9/6 -> Terminator78/1
  CIC Compiler 4.0 9/7 -> Terminator79/1
  CIC Compiler 4.0 9/8 -> Terminator80/1
  Gateway Out1/1 -> LPF chan output/2
  Delay/1 -> CIC reset/2(Channel)
  Delay1/1 -> CIC Compiler 4.0 11/1, CIC Compiler 4.0 12/1, CIC Compiler 4.0 3/1, CIC Compiler 4.0 1/1, CIC Compiler 4.0 2/1, CIC Compiler 4.0 4/1, CIC Compiler 4.0 5/1, CIC Compiler 4.0 6/1, CIC Compiler 4.0 7/1, CIC Compiler 4.0 8/1, CIC Compiler 4.0 9/1, CIC Compiler 4.0 10/1
  Delay2/1 -> CIC Compiler 4.0 12/2
  Delay3/1 -> CIC Compiler 4.0 11/2
  Delay13/1 -> CIC Compiler 4.0 3/2
  Delay14/1 -> CIC Compiler 4.0 1/2
  Delay4/1 -> CIC Compiler 4.0 2/2
  Delay5/1 -> CIC Compiler 4.0 4/2
  Delay6/1 -> CIC Compiler 4.0 5/2
  Delay7/1 -> CIC Compiler 4.0 10/2
  Delay9/1 -> CIC Compiler 4.0 9/2
  Delay8/1 -> CIC Compiler 4.0 8/2
  Delay10/1 -> CIC Compiler 4.0 7/2
  Delay15/1 -> CIC Compiler 4.0 6/2

== system CryoDetXray/DspCore/AdcDac 0/Amplitudes ==
  note: tvalid
  note: Channel #
  note: Sig+
  note: Sig-
  note: Ref+
  note: Ref
  note: Sig
  note: Ref-
  In2 : Inport
  Ampl Scope : Scope  NumInputPorts=5
  Bus Creator : BusCreator  Inputs=3
  Bus Selector1 : BusSelector  OutputSignals=channel&tvalid,I&Qlpf
  Bus Selector2 : BusSelector  OutputSignals=channel,tvalid
  CORDIC 6.0 {,1..4} (5 alike) : xbsIndex_r4/CORDIC 6.0   functional_selection=Translate  architectural_configuration=Parallel  pipelining_mode=Optimal  data_format=SignedFraction  phase_format=Scaled_Radians  input_width=24  output_width=16  round_mode=Truncate  iterations=0  precision=0  compensation_scaling=Embedded_Multiplier  coarse_rotation=on  aclken=off  aresetn=off  out_tready=off  cartesian_has_tuser=off  cartesian_has_tlast=off  cartesian_tuser_width=1  phase_has_tuser=off  phase_has_tlast=off  phase_tuser_width=1  out_tlast_behv=Null  flow_control=Blocking  optimize_goal=Performance  trim_axipin_name=on  simulation_type=hybrid_sim  simulation_model=sysgen:cordic_v6_0  data_path_portlist={'s_axis_cartesian_tdata_imag', 's_axis_cartesian_tdata_real', 's_axis_phase_tdata_phase', 'm_axis_dout_tdata_imag', 'm_axis_dout_tdata_real', 'm_axis_dout_tdata_phase','m_axis_dout_tdata'}  ip_name=CORDIC  ip_version=6.0  dsptool_ready=true  ipcore_usecache=true  ipcore_useipmodelcache=true  wrapper_available=true  port_translation_map={ 'aclken' => 'en', 'aresetn' => 'rst' }  block_type=cordic_v6_0
      settings: infoedit=CORDIC 6.0
  CORDIC 6.0 5 : xbsIndex_r4/CORDIC 6.0   functional_selection=Translate  architectural_configuration=Parallel  pipelining_mode=Optimal  data_format=SignedFraction  phase_format=Scaled_Radians  input_width=24  output_width=16  round_mode=Truncate  iterations=0  precision=0  compensation_scaling=Embedded_Multiplier  coarse_rotation=on  aclken=off  aresetn=off  out_tready=off  cartesian_has_tuser=on  cartesian_has_tlast=off  cartesian_tuser_width=1  phase_has_tuser=off  phase_has_tlast=off  phase_tuser_width=1  out_tlast_behv=Null  flow_control=Blocking  optimize_goal=Performance  trim_axipin_name=on  simulation_type=hybrid_sim  simulation_model=sysgen:cordic_v6_0  data_path_portlist={'s_axis_cartesian_tdata_imag', 's_axis_cartesian_tdata_real', 's_axis_phase_tdata_phase', 'm_axis_dout_tdata_imag', 'm_axis_dout_tdata_real', 'm_axis_dout_tdata_phase','m_axis_dout_tdata'}  ip_name=CORDIC  ip_version=6.0  dsptool_ready=true  ipcore_usecache=true  ipcore_useipmodelcache=true  wrapper_available=true  port_translation_map={ 'aclken' => 'en', 'aresetn' => 'rst' }  block_type=cordic_v6_0
      settings: infoedit=CORDIC 6.0
  Constant : xbsIndex_r4/Constant  const=1  gui_display_data_type=Boolean  arith_type=Boolean  n_bits=16  bin_pt=14  preci_type=Single  exp_width=8  frac_width=24  explicit_period=off  period=1  equ=P=C  opselect=C  inp2=PCIN>>17  opr=+  inp1=P  carry=CIN  dbl_ovrd=off  block_type=constant
  Delay : xbsIndex_r4/Delay  rst=off  infoeditControl=Selection of Reset will increase slice count due to use of real FFs and instead of SRLs  en=off  latency=28  reg_retiming=off  dbl_ovrd=off  block_type=delay
  Delay1 : xbsIndex_r4/Delay  rst=off  infoeditControl=Selection of Reset will increase slice count due to use of real FFs and instead of SRLs  en=off  latency=28  reg_retiming=off  dbl_ovrd=off  block_type=delay
  Demux{1,13,15..18} (6 alike) : Demux  Outputs=2
  Demux14 : Demux  Outputs=6
  Gateway Out{,1..8} (9 alike) : xbsIndex_r4/Gateway Out  inherit_from_input=off  hdl_port=off  rows=1  columns=1  UseAsDAC=off  DACChannel='1'  interface=None  automatic_assignment=on  address_offset=hex2dec('00')  intf_name=''  intf_description=''  timing_constraint=None  locs_specified=off  LOCs={}  io_standard={}  block_type=gatewayout
  Mux : Mux  Inputs=6
  Mux1 : Mux  Inputs=3
  Mux2 : Mux  Inputs=2
  Mux3 : Mux  Inputs=2
  Reinterpret{,1..11} (12 alike) : xbsIndex_r4/Reinterpret  force_arith_type=off  arith_type=Unsigned  force_bin_pt=on  bin_pt=22  block_type=reinterpret
  Terminator{,1..17} (18 alike) : Terminator
  tag scope: AmplBus=global
  wires:
  Demux14/2 -> Demux13/1
  Demux14/3 -> Demux15/1
  Demux14/5 -> Demux17/1
  Demux14/6 -> Demux18/1
  Bus Selector1/2 -> Demux14/1  "<I&Qlpf>"
  In2/1 -> Bus Selector1/1
  Demux14/4 -> Demux16/1
  Bus Selector2/1 -> CORDIC 6.0 5/4, Delay/1  "<channel>"
  Bus Selector1/1 -> Bus Selector2/1  "<channel&tvalid>"
  Demux14/1 -> Demux1/1
  Demux1/2 -> Reinterpret1/1
  Demux1/1 -> Reinterpret/1
  Demux18/1 -> Reinterpret10/1
  Demux18/2 -> Reinterpret11/1
  Demux17/1 -> Reinterpret8/1
  Demux17/2 -> Reinterpret9/1
  Demux16/1 -> Reinterpret6/1
  Demux16/2 -> Reinterpret7/1
  Demux15/1 -> Reinterpret4/1
  Demux15/2 -> Reinterpret5/1
  Demux13/1 -> Reinterpret2/1
  Demux13/2 -> Reinterpret3/1
  Constant/1 -> CORDIC 6.0 1/1, CORDIC 6.0 2/1, CORDIC 6.0 3/1, CORDIC 6.0 4/1, CORDIC 6.0 5/1, "CORDIC 6.0 "/1
  Bus Selector2/2 -> Delay1/1  "<tvalid>"
  Delay/1 -> Gateway Out/1, Bus Creator/1  "channel"
  Delay1/1 -> Gateway Out1/1, Bus Creator/2  "tvalid"
  "CORDIC 6.0 "/4 -> Gateway Out2/1, Mux/1
  CORDIC 6.0 1/4 -> Mux/2, Gateway Out3/1
  CORDIC 6.0 2/4 -> Gateway Out4/1, Mux/3
  CORDIC 6.0 3/4 -> Gateway Out5/1, Mux/4
  CORDIC 6.0 4/4 -> Gateway Out6/1, Mux/5
  CORDIC 6.0 5/4 -> Gateway Out7/1, Mux/6
  Bus Creator/1 -> [AmplBus]
  Mux/1 -> Bus Creator/3  "Ampls"
  Gateway Out/1 -> Mux1/1
  Gateway Out1/1 -> Mux1/2
  Gateway Out3/1 -> Mux2/1
  Gateway Out4/1 -> Mux2/2
  Mux1/1 -> Ampl Scope/1
  Gateway Out2/1 -> Ampl Scope/2
  Mux2/1 -> Ampl Scope/3
  Gateway Out5/1 -> Ampl Scope/4
  Gateway Out6/1 -> Mux3/1
  Gateway Out7/1 -> Mux3/2
  Mux3/1 -> Ampl Scope/5
  "CORDIC 6.0 "/1 -> Terminator/1
  "CORDIC 6.0 "/2 -> Terminator1/1
  "CORDIC 6.0 "/3 -> Terminator2/1
  CORDIC 6.0 1/1 -> Terminator3/1
  CORDIC 6.0 1/2 -> Terminator4/1
  CORDIC 6.0 1/3 -> Terminator5/1
  CORDIC 6.0 2/1 -> Terminator6/1
  CORDIC 6.0 2/2 -> Terminator7/1
  CORDIC 6.0 2/3 -> Terminator8/1
  CORDIC 6.0 3/1 -> Terminator9/1
  CORDIC 6.0 3/2 -> Terminator10/1
  CORDIC 6.0 3/3 -> Terminator11/1
  CORDIC 6.0 4/1 -> Terminator12/1
  CORDIC 6.0 4/2 -> Terminator13/1
  CORDIC 6.0 4/3 -> Terminator14/1
  CORDIC 6.0 5/1 -> Terminator15/1
  CORDIC 6.0 5/2 -> Terminator16/1
  CORDIC 6.0 5/3 -> Terminator17/1
  CORDIC 6.0 5/5 -> Gateway Out8/1
  Gateway Out8/1 -> Mux1/3
  Reinterpret/1 -> "CORDIC 6.0 "/2
  Reinterpret1/1 -> "CORDIC 6.0 "/3
  Reinterpret2/1 -> CORDIC 6.0 1/2
  Reinterpret3/1 -> CORDIC 6.0 1/3
  Reinterpret4/1 -> CORDIC 6.0 2/2
  Reinterpret5/1 -> CORDIC 6.0 2/3
  Reinterpret6/1 -> CORDIC 6.0 3/2
  Reinterpret7/1 -> CORDIC 6.0 3/3
  Reinterpret8/1 -> CORDIC 6.0 4/2
  Reinterpret9/1 -> CORDIC 6.0 4/3
  Reinterpret10/1 -> CORDIC 6.0 5/2
  Reinterpret11/1 -> CORDIC 6.0 5/3
